simulink model "MinSegMotor_n4SID"  (R2024a)
settings: Solver=FixedStepDiscrete  StartTime=0.0  StopTime=60  FixedStep=1/500  RelTol=1e-3  EnableMultiTasking=on
PostLoadFcn:
  | try,
  | codertarget.arduinobase.registry.setBaudRate(gcs,115200)
  | disp('baud rate set to 115200 for external mode hardware serial')
  | baudrate='set_to_115200'
  | catch
  | disp('baud rate setting not needed in this version')
  | end
values from neighbouring files (symbols this model uses):
  s = tf('s')    [Q0_placement.m]    (also in signal_reconstruction_fractional_simulink.m = stairs(t_lin_cs, err_IIR(3,:)); signal_reconstruction_offline.m = stairs(t_inter,err_IIR(3,:)); signal_reconstruction_online.m = stairs(t_fs,y_w(2,:)))
libraries: dspsrcs4 x2, MinSegLibrary_M2V5 x2, slctrl_signal x2
settings Model: SimulationMode=external  ExtModeTrigDuration=2  Creator=Alec  LastModifiedBy=tpjch
settings SolverCC: AlgebraicLoopSolver=TrustRegion
settings DataIOCC: LimitDataPoints=on  SaveFormat=Array  ReturnWorkspaceOutputs=off
settings OptimizationCC: EnhancedBackFolding=on  PassReuseOutputArgsThreshold=0  ExpressionDepthLimit=2147483647  MaxStackSize=64  OptimizeBlockOrder=speed  DifferentSizesBufferReuse=on  OptimizationCustomize=off
settings DebuggingCC: UnderspecifiedInitializationDetection=Classic  MergeDetectMultiDrivingBlocksExec=none  MultiTaskRateTransMsg=warning  ParameterTunabilityLossMsg=error  UnconnectedInputMsg=warning  UnconnectedOutputMsg=warning  UnconnectedLineMsg=warning  StateNameClashWarn=warning  SFUnexpectedBacktrackingDiag=warning  SFNoUnconditionalDefaultTransitionDiag=warning  SFExecutionAtInitializationDiag=none  ArithmeticOperatorsInVariantConditions=warning
settings HardwareCC: ProdBitPerInt=16  ProdBitPerPointer=16  ProdBitPerSizeT=16  ProdBitPerPtrDiffT=16  ProdLargestAtomicFloat=None  ProdWordSize=8  ProdHWDeviceType=Atmel->AVR  UseEmbeddedCoderFeatures=off  UseSimulinkCoderFeatures=off
settings ModelReferenceCC: PropagateSignalLabelsOutOfModel=off
settings SFSimCC: SimUseLocalCustomCode=off  MATLABDynamicMemAlloc=off  CustomCodeUndefinedFunction=UseInterfaceOnly
settings RTWCC: Description=Embedded Coder  SystemTargetFile=ert.tlc  HardwareBoard=Arduino Mega 2560  TemplateMakefile=ert_default_tmf  RTWVerbose=off  RTWUseLocalCustomCode=off  Toolchain=Arduino AVR  BuildConfiguration=Faster Runs  GPUComputeCapability=3.5
settings CodeAppCC: ForceParamTrailComments=on  OperatorAnnotations=on  MangleLength=10
settings ERTTargetCC: ERTCustomFileBanners=off  SupportContinuousTime=on  SupportNonInlinedSFcns=on  RemoveResetFunc=off  SupportVariableSizeSignals=on  ModelStepFunctionPrototypeControlCompliant=off  ExtMode=on  ExtModeTransport=3  ExtModeStaticAlloc=on  ExtModeAutomaticAllocSize=off  ExtModeStaticAllocSize=2048  ExtModeMexFile=ext_xcp  ExtModeMexArgs=0 6 115200  ExtModeIntrfLevel=Level2 - Open  ERTSrcFileBannerTemplate=codertarget_code_template.cgt  ERTHdrFileBannerTemplate=codertarget_code_template.cgt  ERTDataSrcFileTemplate=codertarget_code_template.cgt  ERTDataHdrFileTemplate=codertarget_code_template.cgt
settings ConfigComp: CovMetricSettings=dw  CovSaveCumulativeToWorkspaceVar=on  CovSaveSingleToWorkspaceVar=on  CovExternalEMLEnable=off

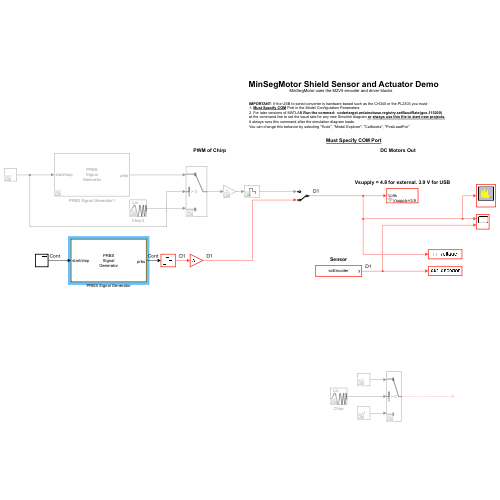
[thumbnail: Simulink's stored preview of the top-level diagram]
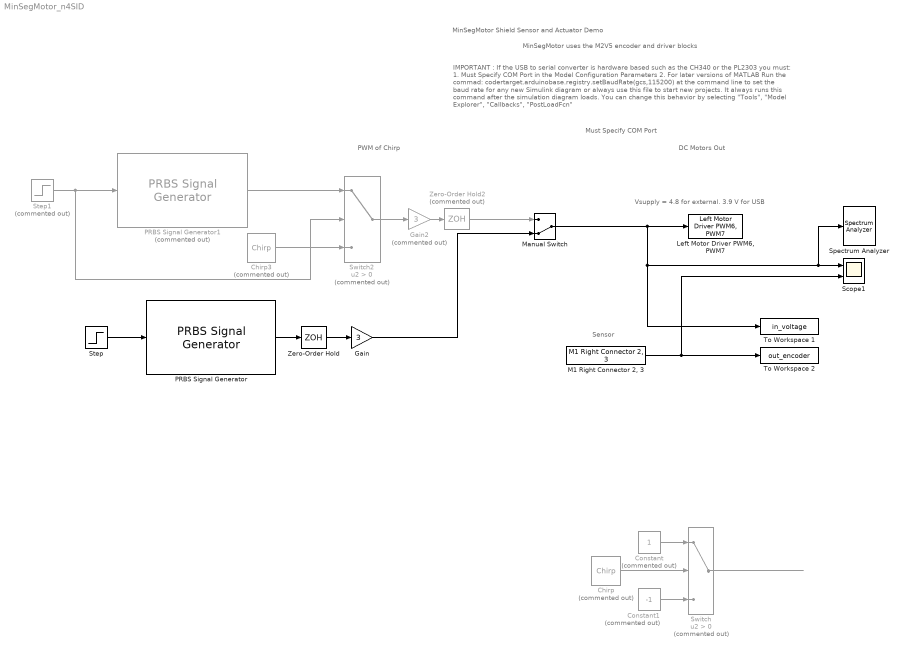
== system MinSegMotor_n4SID ==
  note: MinSegMotor uses the M2V5 encoder and driver blocks
  note: IMPORTANT : If the USB to serial converter is hardware based such as the CH340 or the PL2303 you must:
      | 1. Must Specify COM Port in the Model Configuration Parameters
      | 2. For later versions of MATLAB Run the commad: codertarget.arduinobase.registry.setBaudRate(gcs,115200)
      | at the command line to set the baud rate for any new Simulink diagram or always use this file to start new projects.
      | It always runs this command after the simulation diagram loads.
      | You can change this behavior by selecting "Tools", "Model Explorer", "Callbacks", "PostLoadFcn"
  note: Must Specify COM Port
  note: DC Motors Out
  note: Sensor
  note: MinSegMotor Shield Sensor and Actuator Demo
  note: PWM of Chirp
  note: Vsupply = 4.8 for external. 3.9 V for USB
  Chirp : dspsrcs4/Chirp  Commented=on  sweep=Linear  mode=Unidirectional  f0=0.01  f1=7  t1=15  Tsweep=15  phase=0  Ts=1/500  spf=1  datatype=single  OutputFrames=off
  Chirp3 : dspsrcs4/Chirp  Commented=on  sweep=Linear  mode=Unidirectional  f0=0.1  f1=5  t1=150  Tsweep=150  phase=0  Ts=1/500  spf=1  datatype=double  OutputFrames=off
  Constant : Constant  Commented=on
  Constant1 : Constant  Commented=on  Value=-1
  Gain : Gain  Gain=3
  Gain2 : Gain  Commented=on  Gain=3
  "Left Motor Driver PWM6, PWM7" : MinSegLibrary_M2V5/Left Motor Driver PWM6, PWM7  Vsupply=3.9  PWMoffset=0
  "M1 Right Connector 2, 3" : MinSegLibrary_M2V5/M1 Right Connector 2, 3  Encoder=0  PinA=2  PinB=3
  Manual Switch : ManualSwitch  CurrentSetting=0
  PRBS Signal Generator : slctrl_signal/PRBS Signal Generator  DiscreteTs=1/500  BlockDataType=double  SignalSource=Block parameters  Frequencies=[0.5 1 2]  FreqUnits=rad/s  Amplitudes=2  NumOfFreq=3  NumOfPRBSPeriod=1  UseAutogenNumOfPRBSPeriod=off  PRBSSignalOrder=15  UseAutogenPRBSSignalOrder=off  UseExternalTs=off  CompiledTsChoice=InternalTs
      settings: LibrarySourceBlock=slctrlblks/Signal Generation/PRBS Signal Generator
  PRBS Signal Generator1 : slctrl_signal/PRBS Signal Generator  Commented=on  DiscreteTs=1/500  BlockDataType=double  SignalSource=Block parameters  Frequencies=[0.5 1 2]  FreqUnits=rad/s  Amplitudes=2  NumOfFreq=3  NumOfPRBSPeriod=6  UseAutogenNumOfPRBSPeriod=off  PRBSSignalOrder=15  UseAutogenPRBSSignalOrder=off  UseExternalTs=off  CompiledTsChoice=InternalTs
      settings: LibrarySourceBlock=slctrlblks/Signal Generation/PRBS Signal Generator
  Scope1 : Scope  NumInputPorts=2
  Spectrum Analyzer : SpectrumAnalyzer  WindowPosition=[-1535.000000,-482.000000,638.000000,640.000000,]  Visible=on  ScopeFrameLocation=window  Span=500  StartFrequency=-250  StopFrequency=250  YLimits=[-4.939477243837333,17.176180062473115]  ColorLimits=[-80 20]  ShowLegend=on  SelectedToolstripTab=spectrumAnalyzerToolstrip.spectralMaskTab  AllowFFTLengthLessThanSamplesPerUpdate=on
  Step : Step  Time=0.1  SampleTime=0
  Step1 : Step  Commented=on  Time=150  SampleTime=1/500
  Switch : Switch  Commented=on  Criteria=u2 > Threshold  SaturateOnIntegerOverflow=off  InputSameDT=off
  Switch2 : Switch  Commented=on  Criteria=u2 > Threshold  SaturateOnIntegerOverflow=off  InputSameDT=off
  To Workspace 1 : ToWorkspace  VariableName=in_voltage  SaveFormat=Structure With Time  SampleTime=-1
      settings: MaxDataPoints=Inf
  To Workspace 2 : ToWorkspace  VariableName=out_encoder  SaveFormat=Structure With Time  SampleTime=-1
      settings: MaxDataPoints=Inf
  Zero-Order Hold : ZeroOrderHold  SampleTime=1/500
  Zero-Order Hold2 : ZeroOrderHold  Commented=on  SampleTime=1/500
  wires:
  "M1 Right Connector 2, 3"/1 -> Scope1/2, To Workspace 2/1
  Manual Switch/1 -> To Workspace 1/1, Spectrum Analyzer/1, Scope1/1, "Left Motor Driver PWM6, PWM7"/1
  Switch/1 -> ?
  Chirp/1 -> Switch/2
  Constant1/1 -> Switch/3
  Constant/1 -> Switch/1
  PRBS Signal Generator1/1 -> Switch2/1
  Chirp3/1 -> Switch2/3
  Switch2/1 -> Gain2/1
  Step1/1 -> Switch2/2, PRBS Signal Generator1/1
  Gain/1 -> Manual Switch/2
  Step/1 -> PRBS Signal Generator/1
  PRBS Signal Generator/1 -> Zero-Order Hold/1
  Zero-Order Hold/1 -> Gain/1
  Zero-Order Hold2/1 -> Manual Switch/1
  Gain2/1 -> Zero-Order Hold2/1
